simulink model "dVRK_RDOBS"  (Simulink 8.5)
settings: Solver=ode4  StartTime=0.0  StopTime=length(Tm)/1000  FixedStep=0.001  RelTol=1e-3
libraries: neural x630
(part 12 of 14)

== system dVRK_RDOBS/Joint 5 NN Dyn Ident/Layer 2/Delays 1 ==
  "p{2}" : Inport  PortDimensions=100  SampleTime=0.001
      mask Display: e = 0.06;c1 = [120 230 180]/255;c2 = ([120 230 180]+0)/(256+128);c3 = ([120 230 180]+128)/(256+128);patch([0 1 1 0],[0 0 1 1],c1);patch([0 1 1 1-e 1-e 0+e],[0 0 1 1-e 0+e 0+e],c2);patch([0 0 1 1-e 0+e 0+e],[0 1 1 1-e 1-e 0+e],c3);plot([0 1 1 0 0],[0 0 1 1 0]);
  mux : Mux  Inputs=1
      mask Display: e = 0.06;c1 = [120 150 230]/255;c2 = ([120 150 230]+0)/383;c3 = ([120 150 230]+128)/383;patch([0 1 1 0],[0 0 1 1],c1);patch([0 1 1 1-e 1-e 0+e],[0 0 1 1-e 0+e 0+e],c2);patch([0 0 1 1-e 0+e 0+e],[0 1 1 1-e 1-e 0+e],c3);plot([0 1 1 0 0],[0 0 1 1 0]);disp('Mux')
  "pd{2,1}" : Outport
      mask Display: e = 0.06;c1 = [120 230 180]/255;c2 = ([120 230 180]+0)/(256+128);c3 = ([120 230 180]+128)/(256+128);patch([0 1 1 0],[0 0 1 1],c1);patch([0 1 1 1-e 1-e 0+e],[0 0 1 1-e 0+e 0+e],c2);patch([0 0 1 1-e 0+e 0+e],[0 1 1 1-e 1-e 0+e],c3);plot([0 1 1 0 0],[0 0 1 1 0]);
  wires:
  "p{2}"/1 -> mux/1
  mux/1 -> "pd{2,1}"/1

== system dVRK_RDOBS/Joint 5 NN Dyn Ident/Layer 2/LW{2,1} ==
  "ad{2,1}" : Inport  PortDimensions=100  SampleTime=0.001
      mask Display: e = 0.06;c1 = [120 230 180]/255;c2 = ([120 230 180]+0)/(256+128);c3 = ([120 230 180]+128)/(256+128);patch([0 1 1 0],[0 0 1 1],c1);patch([0 1 1 1-e 1-e 0+e],[0 0 1 1-e 0+e 0+e],c2);patch([0 0 1 1-e 0+e 0+e],[0 1 1 1-e 1-e 0+e],c3);plot([0 1 1 0 0],[0 0 1 1 0]);
  "IW{2,1}(1,:)'" : Constant  Value=[-1.1672418928091097;-0.14421324438722372;6.2239981585431252;-2.8741602007509606;-5.4356613470483222;1.9678281949385299;-0.23938405238385832;-2.6383812591018434;-3.5652578889542688;-8.2309757533284209;0.85169963962632078;7.4932720408412941;-0.46031768460312161;1.195847101057292;1.1322437741166615;-0.11720262683794228;-0.21120968079591645;0.83271962002044997;0.59386099630981004;-0.40541118465511689;-1.7365342080898591;-0.31459080435607273;-0.8152045317005332;-3.4008642601896359;-3.3106106454499811;-1.9806876508457258;-4.2579582871517792;10.58716428454113;0.45385858625548509;-0.15301304704509822;0.23665439770815422;0.5313501044208313;-0.15496589850425588;-0.15126231297284223;0.28872615715724226;0.10577958645601987;-3.7813251528875749;0.45612416106802151;0.90140899063906665;-0.17679622630505953;-0.27354310816088312;-3.4106914135506639;-0.13401966720633196;0.64524418068967937;1.1752193371187065;0.93027048292630932;-1.7495546147501759;-0.23102935076563863;0.14659508107199756;7.292145470139423;-0.27935441175119469;-0.2775726741041733;0.1699099514215307;0.27506024729466738;0.38081798243533621;-0.65254017215642812;0.15065395784279545;5.7117709517805872;-0.91445932568066635;-0.24385826192119428;-0.43198231268904569;0.17915796822619429;-1.3352224723681223;-0.70202746301398711;-5.1404369512278478;-0.42829712467656772;0.45426754824639631;0.12279430000972918;1.2392242171119188;-0.97879758326535671;-0.21196197737226832;0.21720920399844593;-2.7738381016964313;3.6794858004324142;0.71846140868479125;-3.0621358470550062;0.13179686588718195;0.16060456017020308;-0.24243430096056559;3.5284178880830859;3.8987017357872604;0.31330001134997709;0.1839128990637755;4.3608496177853358;-0.10074520006827875;-4.2193061954106046;4.0814479553958671;1.943440916552212;-1.6042139408525298;3.8507046005661301;4.6744571998978284;-0.78103343948630011;0.14170590835153327;0.27874804045227586;-10.283466293485757;1.0506803309724702;0.077647377926496799;-0.09816564485368641;4.3259947650364552;-0.3381856818999206]
      mask Display: e = 0.06;c1 = [120 150 230]/255;c2 = ([120 150 230]+0)/383;c3 = ([120 150 230]+128)/383;patch([0 1 1 0],[0 0 1 1],c1);patch([0 1 1 1-e 1-e 0+e],[0 0 1 1-e 0+e 0+e],c2);patch([0 0 1 1-e 0+e 0+e],[0 1 1 1-e 1-e 0+e],c3);plot([0 1 1 0 0],[0 0 1 1 0]);disp('weights');
  Mux : Mux  Inputs=1
      mask Display: e = 0.06;c1 = [120 150 230]/255;c2 = ([120 150 230]+0)/383;c3 = ([120 150 230]+128)/383;patch([0 1 1 0],[0 0 1 1],c1);patch([0 1 1 1-e 1-e 0+e],[0 0 1 1-e 0+e 0+e],c2);patch([0 0 1 1-e 0+e 0+e],[0 1 1 1-e 1-e 0+e],c3);plot([0 1 1 0 0],[0 0 1 1 0]);disp('Mux');
  dotprod1 : neural/Weight Functions/dotprod
  "lz{2,1}" : Outport
      mask Display: e = 0.06;c1 = [120 230 180]/255;c2 = ([120 230 180]+0)/(256+128);c3 = ([120 230 180]+128)/(256+128);patch([0 1 1 0],[0 0 1 1],c1);patch([0 1 1 1-e 1-e 0+e],[0 0 1 1-e 0+e 0+e],c2);patch([0 0 1 1-e 0+e 0+e],[0 1 1 1-e 1-e 0+e],c3);plot([0 1 1 0 0],[0 0 1 1 0]);
  wires:
  "IW{2,1}(1,:)'"/1 -> dotprod1/1
  "ad{2,1}"/1 -> dotprod1/2
  dotprod1/1 -> Mux/1
  Mux/1 -> "lz{2,1}"/1

== system dVRK_RDOBS/Joint 6 NN Dyn Ident/Layer 1/Delays 1 ==
  "p{1}" : Inport  PortDimensions=12  SampleTime=0.001
      mask Display: e = 0.06;c1 = [120 230 180]/255;c2 = ([120 230 180]+0)/(256+128);c3 = ([120 230 180]+128)/(256+128);patch([0 1 1 0],[0 0 1 1],c1);patch([0 1 1 1-e 1-e 0+e],[0 0 1 1-e 0+e 0+e],c2);patch([0 0 1 1-e 0+e 0+e],[0 1 1 1-e 1-e 0+e],c3);plot([0 1 1 0 0],[0 0 1 1 0]);
  mux : Mux  Inputs=1
      mask Display: e = 0.06;c1 = [120 150 230]/255;c2 = ([120 150 230]+0)/383;c3 = ([120 150 230]+128)/383;patch([0 1 1 0],[0 0 1 1],c1);patch([0 1 1 1-e 1-e 0+e],[0 0 1 1-e 0+e 0+e],c2);patch([0 0 1 1-e 0+e 0+e],[0 1 1 1-e 1-e 0+e],c3);plot([0 1 1 0 0],[0 0 1 1 0]);disp('Mux')
  "pd{1,1}" : Outport
      mask Display: e = 0.06;c1 = [120 230 180]/255;c2 = ([120 230 180]+0)/(256+128);c3 = ([120 230 180]+128)/(256+128);patch([0 1 1 0],[0 0 1 1],c1);patch([0 1 1 1-e 1-e 0+e],[0 0 1 1-e 0+e 0+e],c2);patch([0 0 1 1-e 0+e 0+e],[0 1 1 1-e 1-e 0+e],c3);plot([0 1 1 0 0],[0 0 1 1 0]);
  wires:
  "p{1}"/1 -> mux/1
  mux/1 -> "pd{1,1}"/1
